simulink model "ksrbl_4k4t_hdtrig"  (Simulink 6.2)
settings: Solver=ode45  StartTime=0.0  StopTime=20000  RelTol=1e-3
libraries: xbsIndex_r3 x1214, casper_library x120, xps_library x20
(part 26 of 26)

== system ksrbl_4k4t_hdtrig/fft_wideband_real/fft_biplex_real_4x0/biplex_core/fft_stage_9/butterfly_direct/twiddle ==
  a : Inport  Port=1  LatchInput=off
  b : Inport  Port=2  LatchInput=off
  sync : Inport  Port=3  LatchInput=off
  twiddle_general_3mult : casper_library/FFTs/Twiddle/twiddle_general_3mult  Coeffs="[1+0i           6.1232e-017-1i               0.70711-0.70711i        -0.70711-0.70711i         0.92388-0.38268i        -0.38268-0.92388i         0.38268-0.92388i        -0.92388-0.38268i         0.98079-0.19509i        -0.19509-0.98079i         0.55557-0.83147i        -0.83147-0.55557i         0.83147-0.55557i        -0.55557-0.83147i         0.19509-0.98079i        -0.98079-0.19509i         0.99518-0.098017i      -0.098017-0.99518i         0.63439-0.77301i        -0.77301-0.63439i         0.88192-0.4714i          -0.4714-0.88192i         0.29028-0.95694i        -0.95694-0.29028i         0.95694-0.29028i        -0.29028-0.95694i          0.4714-0.88192i        -0.88192-0.4714i          0.77301-0.63439i        -0.63439-0.77301i        0.098017-0.99518i        -0.99518-0.098017i         0.9988-0.049068i      -0.049068-0.9988i          0.67156-0.74095i        -0.74095-0.67156i         0.90399-0.42756i        -0.42756-0.90399i         0.33689-0.94154i        -0.94154-0.33689i         0.97003-0.24298i        -0.24298-0.97003i          0.5141-0.85773i        -0.85773-0.5141i          0.80321-0.5957i          -0.5957-0.80321i         0.14673-0.98918i        -0.98918-0.14673i         0.98918-0.14673i        -0.14673-0.98918i          0.5957-0.80321i        -0.80321-0.5957i          0.85773-0.5141i          -0.5141-0.85773i         0.24298-0.97003i        -0.97003-0.24298i         0.94154-0.33689i        -0.33689-0.94154i         0.42756-0.90399i        -0.90399-0.42756i         0.74095-0.67156i        -0.67156-0.74095i        0.049068-0.9988i          -0.9988-0.049068i         0.9997-0.024541i      -0.024541-0.9997i          0.68954-0.72425i        -0.72425-0.68954i         0.91421-0.40524i        -0.40524-0.91421i          0.3599-0.93299i        -0.93299-0.3599i           0.9757-0.2191i          -0.2191-0.9757i            0.535-0.84485i        -0.84485-0.535i           0.81758-0.57581i        -0.57581-0.81758i         0.17096-0.98528i        -0.98528-0.17096i         0.99248-0.12241i        -0.12241-0.99248i         0.61523-0.78835i        -0.78835-0.61523i         0.87009-0.4929i          -0.4929-0.87009i         0.26671-0.96378i        -0.96378-0.26671i         0.94953-0.31368i        -0.31368-0.94953i         0.44961-0.89322i        -0.89322-0.44961i         0.75721-0.65317i        -0.65317-0.75721i        0.073565-0.99729i        -0.99729-0.073565i        0.99729-0.073565i      -0.073565-0.99729i         0.65317-0.75721i        -0.75721-0.65317i         0.89322-0.44961i        -0.44961-0.89322i         0.31368-0.94953i        -0.94953-0.31368i         0.96378-0.26671i        -0.26671-0.96378i          0.4929-0.87009i        -0.87009-0.4929i          0.78835-0.61523i        -0.61523-0.78835i         0.12241-0.99248i        -0.99248-0.12241i         0.98528-0.17096i        -0.17096-0.98528i         0.57581-0.81758i        -0.81758-0.57581i         0.84485-0.535i            -0.535-0.84485i          0.2191-0.9757i          -0.9757-0.2191i          0.93299-0.3599i          -0.3599-0.93299i         0.40524-0.91421i        -0.91421-0.40524i         0.72425-0.68954i        -0.68954-0.72425i        0.024541-0.9997i          -0.9997-0.024541i        0.99992-0.012272i      -0.012272-0.99992i         0.69838-0.71573i        -0.71573-0.69838i         0.91911-0.39399i        -0.39399-0.91911i         0.37132-0.92851i        -0.92851-0.37132i         0.97832-0.20711i        -0.20711-0.97832i         0.54532-0.83822i        -0.83822-0.54532i         0.82459-0.56573i        -0.56573-0.82459i         0.18304-0.98311i        -0.98311-0.18304i         0.99391-0.11022i        -0.11022-0.99391i         0.62486-0.78074i        -0.78074-0.62486i         0.87607-0.48218i        -0.48218-0.87607i         0.27852-0.96043i        -0.96043-0.27852i         0.95331-0.30201i        -0.30201-0.95331i         0.46054-0.88764i        -0.88764-0.46054i         0.76517-0.64383i        -0.64383-0.76517i        0.085797-0.99631i        -0.99631-0.085797i ...(+2393 chars)   ]"  StepPeriod=1  BitWidth=18  add_latency=4  mult_latency=6  bram_latency=4
  a_re : Outport
  a_im : Outport  Port=2
  bw_re : Outport  Port=3
  bw_im : Outport  Port=4
  sync_out : Outport  Port=5
  wires:
  a/1 -> twiddle_general_3mult/1
  b/1 -> twiddle_general_3mult/2
  sync/1 -> twiddle_general_3mult/3
  twiddle_general_3mult/1 -> a_re/1
  twiddle_general_3mult/2 -> a_im/1
  twiddle_general_3mult/3 -> bw_re/1
  twiddle_general_3mult/4 -> bw_im/1
  twiddle_general_3mult/5 -> sync_out/1
